simulink model "InductionCookerDeploy"  (R2022b)
settings: Solver=FixedStepAuto  StartTime=0.0  StopTime=240  FixedStep=0.1  RelTol=1e-3  EnableMultiTasking=on
libraries: mbedblockslib x7
settings Model: ExtModeTrigDuration=10  Creator=alewi  LastModifiedBy=cristian
settings OptimizationCC: ReuseModelBlockBuffer=on  EnhancedBackFolding=on  PassReuseOutputArgsAs=Individual arguments  ZeroExternalMemoryAtStartup=off  ZeroInternalMemoryAtStartup=off  MaxStackSize=64  OptimizeBlockOrder=speed  DifferentSizesBufferReuse=on  OptimizationCustomize=off  EfficientTunableParamExpr=on
settings DebuggingCC: ParameterTunabilityLossMsg=error
settings HardwareCC: ProdBitPerPointer=32  ProdBitPerSizeT=32  ProdBitPerPtrDiffT=32  ProdLargestAtomicInteger=Long  ProdLargestAtomicFloat=Double  ProdWordSize=32  ProdLongLongMode=on  ProdHWDeviceType=ARM Compatible->ARM Cortex
settings SFSimCC: MATLABDynamicMemAlloc=off
settings RTWCC: Description=Embedded Coder  SystemTargetFile=ert.tlc  HardwareBoard=STM32 Nucleo F401RE  TLCOptions=-aInlineSetEventsForThisBaseRateFcn=TLC_FALSE -aSuppressMultiTaskScheduler=TLC_FALSE -aRateBasedStepFcn=1  TemplateMakefile=ert_default_tmf  Toolchain=GNU Tools for ARM Embedded Processors
settings CodeAppCC: ForceParamTrailComments=on  IgnoreCustomStorageClasses=off  OperatorAnnotations=on  SimulinkDataObjDesc=on  SFDataObjDesc=on  InsertBlockDesc=on
settings ERTTargetCC: ExtModeTransport=3  ExtModeStaticAlloc=on  ExtModeStaticAllocSize=2000  ExtModeMexFile=ext_xcp  ExtModeIntrfLevel=Level2 - Open
settings ConfigComp: CovHTMLOptions=-sRT=1 -sVT=0 -aTS=1 -agT=1 -bRG=1 -bTC=1 -hTR=0 -nFC=0 -nFD=1 -scm=1 -bcm=1 -xEv=0 -xEM=0 -req=1  CovEnableCumulative=off

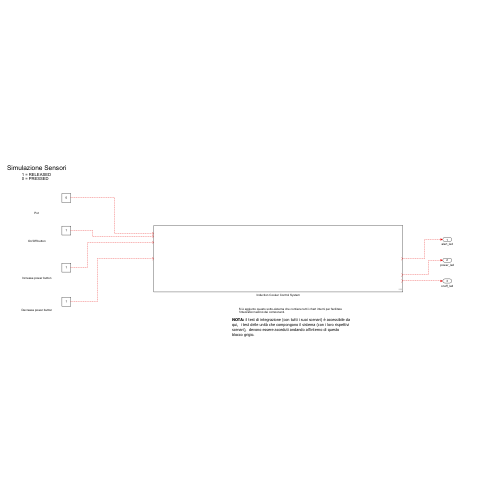
[thumbnail: Simulink's stored preview of the top-level diagram]
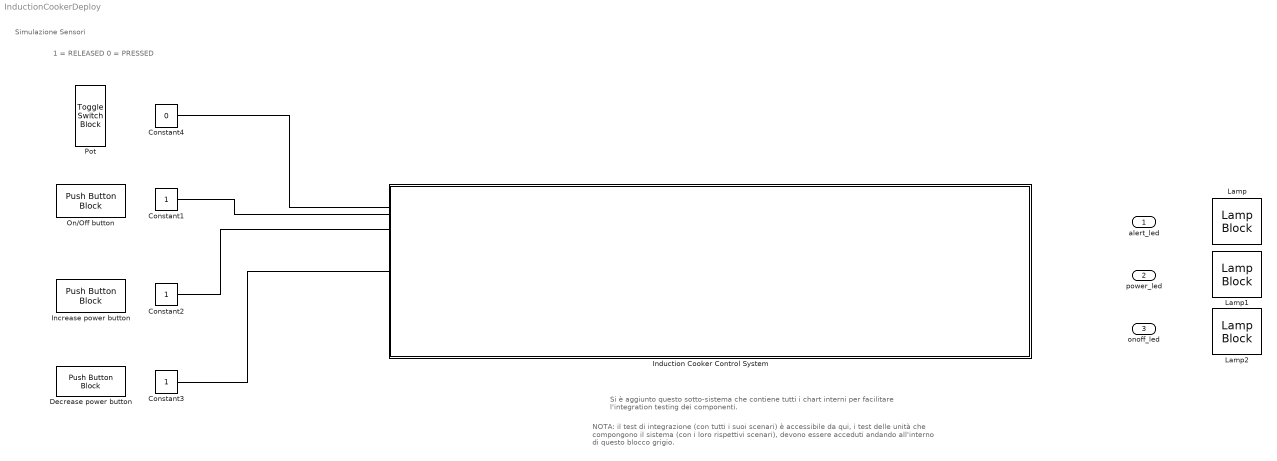
== system InductionCookerDeploy ==
  note: NOTA: il test di integrazione (con tutti i suoi scenari) è accessibile da qui, i test delle unità che compongono il sistema (con i loro rispettivi scenari), devono essere acceduti andando all'interno di questo blocco grigio.
  note: Si è aggiunto questo sotto-sistema che contiene tutti i chart interni per facilitare l'integration testing dei componenti.
  note: 1 = RELEASED
      | 0 = PRESSED
  note: Simulazione Sensori
  Constant1 : Constant  OutDataTypeStr=boolean
  Constant2 : Constant  OutDataTypeStr=boolean
  Constant3 : Constant  OutDataTypeStr=boolean
  Constant4 : Constant  Value=0  OutDataTypeStr=boolean
  Decrease power button : PushButtonBlock  OnValue=0  ButtonType=Latch  OffValue=1.000000
  Increase power button : PushButtonBlock  OnValue=0  ButtonType=Latch  OffValue=1.000000
  Induction Cooker Control System : Subsystem
  Lamp : LampBlock  LabelPosition=Hide
  Lamp1 : LampBlock  LabelPosition=Hide
  Lamp2 : LampBlock  LabelPosition=Hide
  On/Off button : PushButtonBlock  OnValue=0  ButtonType=Latch  IconColor=On  OffValue=1.000000
  Pot : ToggleSwitchBlock
      settings: Values={{'No Pot', 'Pot'}, [1 0]}
  alert_led : Outport
  power_led : Outport  Port=2
  onoff_led : Outport  Port=3
  wires:
  Constant4/1 -> ?
  Constant1/1 -> ?
  Constant2/1 -> ?
  Constant3/1 -> ?
  ? -> alert_led/1
  ? -> power_led/1
  ? -> onoff_led/1

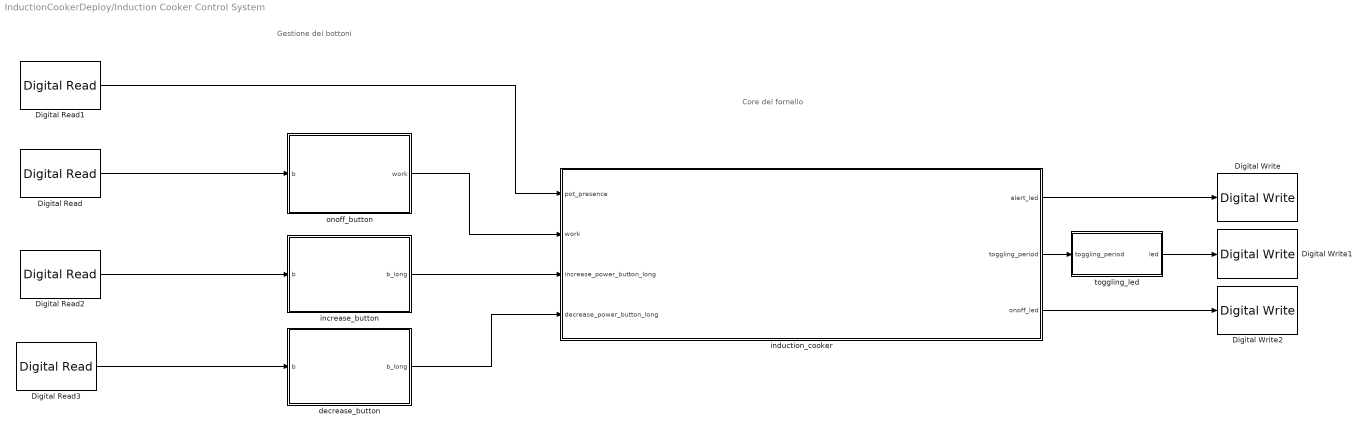
== system InductionCookerDeploy/Induction Cooker Control System ==
  note: Core del fornello
  note: Gestione dei bottoni
  Digital Read : mbedblockslib/Digital Read  Pin=PC_13  Direction=input  SampleTime=-1
      settings: LibrarySourceBlock=stmnucleorootlib/Common/Digital Read
  Digital Read1 : mbedblockslib/Digital Read  Pin=PC_3  Direction=input  SampleTime=-1
      settings: LibrarySourceBlock=stmnucleorootlib/Common/Digital Read
  Digital Read2 : mbedblockslib/Digital Read  Pin=PC_10  Direction=input  SampleTime=-1
      settings: LibrarySourceBlock=stmnucleorootlib/Common/Digital Read
  Digital Read3 : mbedblockslib/Digital Read  Pin=PC_12  Direction=input  SampleTime=-1
      settings: LibrarySourceBlock=stmnucleorootlib/Common/Digital Read
  Digital Write : mbedblockslib/Digital Write  Pin=PA_5  Direction=output
      settings: LibrarySourceBlock=stmnucleorootlib/Common/Digital Write
  Digital Write1 : mbedblockslib/Digital Write  Pin=PA_6  Direction=output
      settings: LibrarySourceBlock=stmnucleorootlib/Common/Digital Write
  Digital Write2 : mbedblockslib/Digital Write  Pin=PA_7  Direction=output
      settings: LibrarySourceBlock=stmnucleorootlib/Common/Digital Write
  decrease_button : Stateflow chart  TreatAsAtomicUnit=on
  increase_button : Stateflow chart  TreatAsAtomicUnit=on
  induction_cooker : Stateflow chart  TreatAsAtomicUnit=on
  onoff_button : Stateflow chart  TreatAsAtomicUnit=on
  toggling_led : Stateflow chart  TreatAsAtomicUnit=on
  wires:
  toggling_led/1(led) -> Digital Write1/1
  Digital Read/1 -> onoff_button/1(b)
  Digital Read1/1 -> induction_cooker/1(pot_presence)
  Digital Read3/1 -> decrease_button/1(b)
  decrease_button/1(b_long) -> induction_cooker/4(decrease_power_button_long)
  induction_cooker/1(alert_led) -> Digital Write/1
  Digital Read2/1 -> increase_button/1(b)
  increase_button/1(b_long) -> induction_cooker/3(increase_power_button_long)
  induction_cooker/3(onoff_led) -> Digital Write2/1
  onoff_button/1(work) -> induction_cooker/2(work)
  induction_cooker/2(toggling_period) -> toggling_led/1(toggling_period)

== stateflow chart InductionCookerDeploy/Induction Cooker Control System/decrease_button ==
  note: Bottone a livelli, la pressione per un numero di secondi pari a DURATION permette di avere un uscita alta in maniera istantanea.
      | Per avere in output un valore PRESSED, è necessare lasciare il bottone e premere tra un output e l'altro.
  state Wait
    en: b_long = RELEASED
  state Pressed
    en: b_long = RELEASED;
    on after(DURATION,sec): b_long = PRESSED
  state LongPressed
    en: b_long = RELEASED
  (default) -> Wait
  Wait -> Pressed : [b == PRESSED]
  Pressed -> Wait [order 1] : [b == RELEASED]
  LongPressed -> Wait : [b == RELEASED]
  Pressed -> LongPressed [order 2] : [b_long == PRESSED && b == PRESSED]
  data: b_long output boolean size=1; PRESSED constant boolean size=1 =0; RELEASED constant boolean size=1 =1; b input boolean size=1; DURATION constant double size=1 =1

== stateflow chart InductionCookerDeploy/Induction Cooker Control System/onoff_button ==
  note: Stato di accensione del bottone onoff
  note: In questo stato il bottone può accendere la macchina
  state INACTIVE
    state Pressed
      en: work = HIGH
    state Wait
      en: work = LOW
    (default) -> INACTIVE.Wait
    INACTIVE.Wait -> INACTIVE.Pressed : [b == PRESSED]
  note: Stato di spegnimento del bottone onoff
  note: In questo stato il bottone può spengere la macchina
  state ACTIVE
    state Wait
      en:
      b_long = RELEASED
    state Pressed
      en:
      b_long = RELEASED;
      on after(DURATION,sec): b_long = PRESSED
    state LongPressed
      en: work = LOW;
    (default) -> ACTIVE.Wait
    ACTIVE.Wait -> ACTIVE.Pressed : [b == PRESSED]
    ACTIVE.Pressed -> ACTIVE.Wait [order 1] : [b == RELEASED]
    ACTIVE.Pressed -> LongPressed [order 2] : [b_long == PRESSED && b == PRESSED]
  note: Se il bottone viene premuto una sola volta, il sistema viene acceso.
      | Se il bottone viene premuto per 1 secondo, il sistema viene spento.
      | Una pressione prolungata senza rilascio del bottone, non causa un alternarsi di accensioni e spegnimenti continui.
  (default) -> INACTIVE
  INACTIVE.Pressed -> ACTIVE : [b == RELEASED]
  LongPressed -> INACTIVE : [b==RELEASED]
  data: PRESSED constant boolean size=1 =0; RELEASED constant boolean size=1 =1; b input boolean size=1; DURATION constant double size=1 =1; b_long local boolean size=1; HIGH constant boolean size=1 =1; LOW constant boolean size=1 =0; work output boolean size=1

== stateflow chart InductionCookerDeploy/Induction Cooker Control System/toggling_led ==
  note: Lo spegnimento ha invece la priorità, appena ho periodo=0 spengo.
  state Off
    en: led = LOW
  state Blink_Off
    en:
    led = LOW
    period = toggling_period
  state Blink_On
    en:
    led = HIGH
    period = toggling_period
  note: L'utilizzo di una variabile di appoggio consente di gestire il caso in cui durante il blinking il periodo viene cambiato. Usando tale variabile, lo stato corrente viene termianto dopo un'attesa pari al vecchio periodo e dal nuovo stato vi sarà la variazione di periodo.
      | Ad esempio, se passo da 1s a 2s, ed attualmente il led è acceso, lo spegnerò terminando l'attesa di 1s e dal prossimo stato l'attesa sarà di 2s.
  (default) -> Off
  Blink_Off -> Off [order 1] : [toggling_period == 0]
  Blink_On -> Off [order 1] : [toggling_period == 0]
  Off -> Blink_On : [toggling_period ~= 0]
  Blink_On -> Blink_Off [order 2] : [after(period,sec)]
  Blink_Off -> Blink_On [order 2] : [after(period,sec)]
  data: toggling_period input double; led output boolean; HIGH constant boolean =1; LOW constant boolean =0; period local

== stateflow chart InductionCookerDeploy/Induction Cooker Control System/induction_cooker ==
  note: Il core del fornello è composto da un chart principale che oscilla tra uno stato ON ed uno stato OFF, a seconda dell'input work che ne indica in che stato di funzionamento deve essere (associato al bottone a livelli di on/off).
  state OFF
    en: onoff_led = LOW, alert_led = LOW,
    current_power = 0, toggling_period = TOGGLING_PERIOD_OFF
  note: Lo stato ON è composto da tre macchine parallele che gestiscono rispettivamente: cambiamento potenza, allarme e blink del led.
  state ON
    state LOGIC [parallel]
      settings: executionOrder=1
      note: In LOGIC, lo stato di ingresso è quello a 0W, in quanto appena accendiamo il fornello esso non è attivo.
          | Quando si riceve l'input di INCREASE o DECREASE button, si transita in uno stato che rappresenta una nuova potenza selezionata, dopo 5 secondi da un passaggio di stato la potenza reale diventerà quella associata allo stato correntemente attivo.
          | Quando una certa potenza viene selezionata, viene aggiornato il periodo di blink del power_led.
      state P0W
        state WAIT
        state SET
          en:
          current_power = 0, toggling_period = TOGGLING_PERIOD_0W
        note: Lo stato che rappresenta 0W gode della particolarità di poter fissare la potenza anche senza attendere i 5s, questo è possibile quando da uno stato gerarchicamente superiore o parallelo viene impostato current_power = 0W. Tale circostanza avviene sia all'avvio in cui non vi è necessità di attendere del tempo prima di impostare la potenza a 0W e sia nel momento in cui scatta l'allarme, in cui si disattiva il fornello istantaneamente.
        (default) -> ON.LOGIC.P0W.WAIT
        ON.LOGIC.P0W.WAIT -> ON.LOGIC.P0W.SET : [after(SET_POWER_PATIENCE,sec) || current_power == 0]
      note: Notiamo che in ogni stato di LOGIC, diverso da 0W, vi è una transizione associata al fatto che la variabile alarm assume valore HIGH, che ci riporta automaticamente nello stato 0W e fissa tale potenza come potenza corrente senza attendere i 10 secondi.
      state P1500W
        state WAIT
        state SET
          en:
          current_power = 1500, toggling_period = TOGGLING_PERIOD_1500W
        (default) -> ON.LOGIC.P1500W.WAIT
        ON.LOGIC.P1500W.WAIT -> ON.LOGIC.P1500W.SET : after(SET_POWER_PATIENCE,sec)
      state P300W
        state WAIT
        state SET
          en:
          current_power = 300, toggling_period = TOGGLING_PERIOD_300W
        (default) -> ON.LOGIC.P300W.WAIT
        ON.LOGIC.P300W.WAIT -> ON.LOGIC.P300W.SET : after(SET_POWER_PATIENCE,sec)
      state P1000W
        state WAIT
        state SET
          en:
          current_power = 1000, toggling_period = TOGGLING_PERIOD_1000W
        (default) -> ON.LOGIC.P1000W.WAIT
        ON.LOGIC.P1000W.WAIT -> ON.LOGIC.P1000W.SET : after(SET_POWER_PATIENCE,sec)
      state P500W
        state WAIT
        state SET
          en:
          current_power = 500, toggling_period = TOGGLING_PERIOD_500W
        (default) -> ON.LOGIC.P500W.WAIT
        ON.LOGIC.P500W.WAIT -> ON.LOGIC.P500W.SET : after(SET_POWER_PATIENCE,sec)
      (default) -> P0W
      P1500W -> P0W [order 2] : [alarm == HIGH]
      P0W -> P300W : [increase_power_button_long == PRESSED && pot_presence == PRESSED]
      P300W -> P0W [order 1] : [(alarm == HIGH) || (decrease_power_button_long == PRESSED && pot_presence == PRESSED)]
      P500W -> P0W [order 3] : [alarm == HIGH]
      P1000W -> P0W [order 3] : [alarm == HIGH]
      P500W -> P300W [order 1] : [decrease_power_button_long == PRESSED && pot_presence == PRESSED]
      P300W -> P500W [order 2] : [increase_power_button_long == PRESSED && pot_presence == PRESSED]
      P1500W -> P1000W [order 1] : [decrease_power_button_long == PRESSED && pot_presence == PRESSED]
      P1000W -> P1500W [order 2] : [increase_power_button_long == PRESSED && pot_presence == PRESSED]
      P500W -> P1000W [order 2] : [increase_power_button_long == PRESSED && pot_presence == PRESSED]
      P1000W -> P500W [order 1] : [decrease_power_button_long == PRESSED && pot_presence == PRESSED]
    state ALARM [parallel]
      settings: executionOrder=2
      state ACTIVE
        state QUIET
          en: alarm = LOW, alert_led = LOW
        state ALARM
          en: alert_led = HIGH
          on after(ALARM_PATIENCE,sec): alarm = HIGH; current_power = 0; toggling_period = TOGGLING_PERIOD_0W; alert_led = LOW;
        (default) -> QUIET
        QUIET -> ON.ALARM.ACTIVE.ALARM : [pot_presence == RELEASED]
        ON.ALARM.ACTIVE.ALARM -> QUIET : [pot_presence == PRESSED]
      state INACTIVE
        en:
        alarm = LOW,
        alert_led = LOW
      (default) -> INACTIVE
      INACTIVE -> ACTIVE : [current_power ~= 0]
      ACTIVE -> INACTIVE : [current_power == 0]
    state TOGGLING_LED [parallel] [commented out]
      note: In ogni stato di LOGIC, che rappresenta una specifica potenza, viene impostato un valore di periodo che indica ogni quanto il power_led (led giallo) lampeggia.
          | Infatti, tale macchina semplicemente rimbalza da uno stato all'altro accendendo e spegnendo il led.
      state LED_OFF [commented out]
        en: power_led=LOW;
      state LED_ON [commented out]
        en: power_led=HIGH;
      (default) -> LED_OFF [commented out]
      LED_OFF -> LED_ON [commented out] : [toggling_period>0 && after(toggling_period,sec)]
      LED_ON -> LED_OFF [commented out] : [after(toggling_period,sec)]
  note: Quando la macchina non è attiva (current_power = 0W), anche l'allarme è inattivo. All'attivazione del fornello corrisponde l'attivazione dell'allarme.
      | Nel momento in cui l'allarme è attivo e rileva una rimozione della pentola passa in uno stato ALARM che accende l'alert_led e dopo 10 secondi di permanenza disattiva il sistema portando LOGIC nello stato 0W, a meno di reinserimento pentola che riporta in uno stato QUIET.
  (default) -> OFF
  OFF -> ON : [work == HIGH]{onoff_led = HIGH}
  ON -> OFF : [work == LOW]
  data: pot_presence input boolean size=1; work input boolean size=1; alarm local boolean size=1; alert_led output boolean size=1; toggling_period output double size=1; onoff_led output boolean size=1; current_power local uint16 size=1; increase_power_button_long input boolean size=1; decrease_power_button_long input boolean size=1; HIGH constant boolean size=1 =1; PRESSED constant boolean size=1 =0; RELEASED constant boolean size=1 =1; LOW constant boolean size=1 =0; ALARM_PATIENCE constant double =10; TOGGLING_PERIOD_0W constant double =0; TOGGLING_PERIOD_300W constant double =2; TOGGLING_PERIOD_500W constant double =1; TOGGLING_PERIOD_1000W constant double =0.5; TOGGLING_PERIOD_1500W constant double =0.25; SET_POWER_PATIENCE local =5; TOGGLING_PERIOD_OFF constant double =0

== stateflow chart InductionCookerDeploy/Induction Cooker Control System/increase_button ==
  note: Bottone a livelli, la pressione per un numero di secondi pari a DURATION permette di avere un uscita alta in maniera istantanea.
      | Per avere in output un valore PRESSED, è necessare lasciare il bottone e premere tra un output e l'altro.
  state Wait
    en: b_long = RELEASED
  state Pressed
    en: b_long = RELEASED;
    on after(DURATION,sec): b_long = PRESSED
  state LongPressed
    en: b_long = RELEASED
  (default) -> Wait
  Wait -> Pressed : [b == PRESSED]
  Pressed -> Wait [order 1] : [b == RELEASED]
  LongPressed -> Wait : [b == RELEASED]
  Pressed -> LongPressed [order 2] : [b_long == PRESSED && b == PRESSED]
  data: b_long output boolean size=1; PRESSED constant boolean size=1 =0; RELEASED constant boolean size=1 =1; b input boolean size=1; DURATION constant double size=1 =1
